simulink model "PWM_block"  (R2020a)
settings: Solver=VariableStepAuto  StartTime=0.0  StopTime=0.002  RelTol=1e-3
libraries: eePwmGenerator x1
settings Model: Creator=Naeem Mohammad  LastModifiedBy=Naeem Mohammad

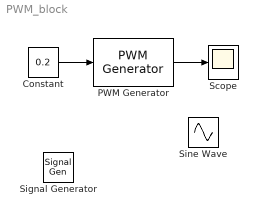
== system PWM_block ==
  Constant : Constant  Value=0.2
  PWM Generator : eePwmGenerator/PWM Generator  CarrCount=Up  Tper=0.001  Ts=5e-5
  Scope : Scope
  Signal Generator : SignalGenerator  WaveForm=square  Units=rad/sec
  Sine Wave : Sin  SampleTime=0
  wires:
  Constant/1 -> PWM Generator/1
  PWM Generator/1 -> Scope/1
